simulink model "HighLevelLowLevel_Manual"  (R2023a)
settings: Solver=FixedStepAuto  StartTime=0.0  StopTime=25  FixedStep=0.0025  RelTol=1e-3
InitFcn:
  | startup
model workspace (MAT data in the model file):
  Cd = 2.24197803e-06
  Ct = 0.00010297
  Ixx = 113600
  Iyy = 113600
  Izz = 22620
  h = 0.05
values from neighbouring files (symbols this model uses):
  B_t = pinv(B)    [startup.m]
  g = 9.806    [startup.m]
  invI = I^-1    [startup.m]
  K_HL = round(K_HL, 6)    [startup.m]
  K_HL_FF = [K_HLtx(1,1), zeros(1,5), K_HLtx(1,2), zeros(1,5), K_HLtx(1,3), zeros(1,5) ... (first row only)    [startup.m]
  K_HL_manual = round(K_HL_manual, 6)    [startup.m]
  l = 0.053336    [startup.m]
  m = 6.2    [startup.m]
  sample_rate = 0.0025    [startup.m]
libraries: simulink_extras x12, matrix_library x8, aerolibanimutils x2, dspmtrx3 x2, shared6dof x1, commchan3 x1
settings Model: Creator=awahm  LastModifiedBy=lachlainm
settings DataIOCC: SaveFormat=StructureWithTime
settings OptimizationCC: DefaultParameterBehavior=Inlined  UseDivisionForNetSlopeComputation=on  GainParamInheritBuiltInType=on  UseFloatMulNetSlope=on  OptimizeBlockIOStorage=off  ZeroExternalMemoryAtStartup=off  ZeroInternalMemoryAtStartup=off  LifeSpan=1  OptimizeDataStoreBuffers=off  BusAssignmentInplaceUpdate=off
settings DebuggingCC: SFUnexpectedBacktrackingDiag=warning  SFNoUnconditionalDefaultTransitionDiag=warning
settings RTWCC: GenerateReport=on  BuildConfiguration=Debug  LaunchReport=on  TargetLang=C++
settings CodeAppCC: ForceParamTrailComments=on  MATLABSourceComments=on  EnableCustomComments=on
settings GRTTargetCC: TargetLangStandard=C++11 (ISO)  CombineSignalStateStructs=on  CodeInterfacePackaging=C++ class  SupportVariableSizeSignals=on  MultiInstanceErrorCode=Warning

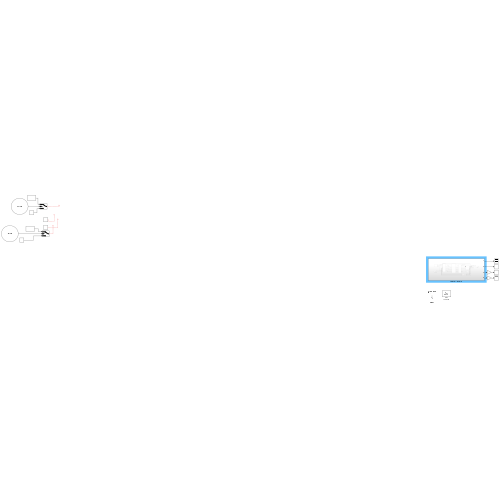
[thumbnail: Simulink's stored preview of the top-level diagram]
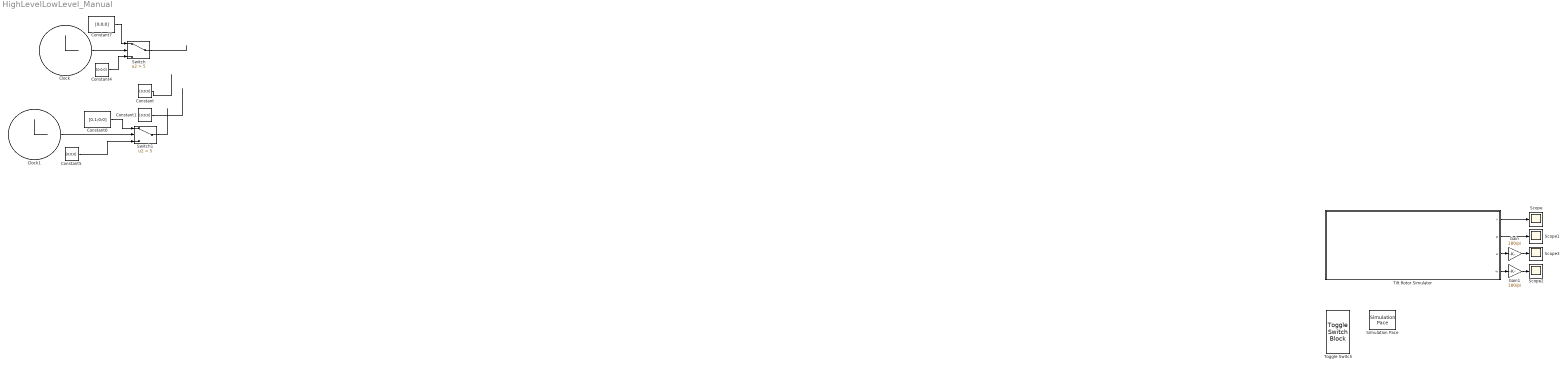
== system HighLevelLowLevel_Manual ==
  Clock : Clock
  Clock1 : Clock
  Constant{,1,4..5,7} (5 alike) : Constant  Value=[0;0;0]
  Constant6 : Constant  Value=[0.1;0;0]
  Gain : Gain  Gain=180/pi
  Gain1 : Gain  Gain=180/pi
  Scope{,1..3} (4 alike) : Scope
  Simulation Pace : aerolibanimutils/Simulation Pace  SimulationPace=1  SleepMode=Auto  OutputPaceError=off  SampleTime=sample_rate
  Switch : Switch  Criteria=u2 > Threshold  Threshold=5  SaturateOnIntegerOverflow=off  InputSameDT=off
  Switch1 : Switch  Criteria=u2 > Threshold  Threshold=5  SaturateOnIntegerOverflow=off  InputSameDT=off
  Tilt Rotor Simulator : Subsystem
  Toggle Switch : ToggleSwitchBlock
      settings: Values={{'Manual', 'Autonomous'}, [0 1]}
  wires:
  Constant/1 -> ?
  Switch1/1 -> ?
  Constant1/1 -> ?
  Clock/1 -> Switch/2
  Constant7/1 -> Switch/1
  Switch/1 -> ?
  Constant4/1 -> Switch/3
  Clock1/1 -> Switch1/2
  Constant6/1 -> Switch1/1
  Constant5/1 -> Switch1/3
  Tilt Rotor Simulator/1(v) -> Scope/1
  Tilt Rotor Simulator/4(w) -> Gain1/1
  Tilt Rotor Simulator/3(a) -> Gain/1
  Tilt Rotor Simulator/2(p) -> Scope1/1
  Gain/1 -> Scope3/1
  Gain1/1 -> Scope2/1

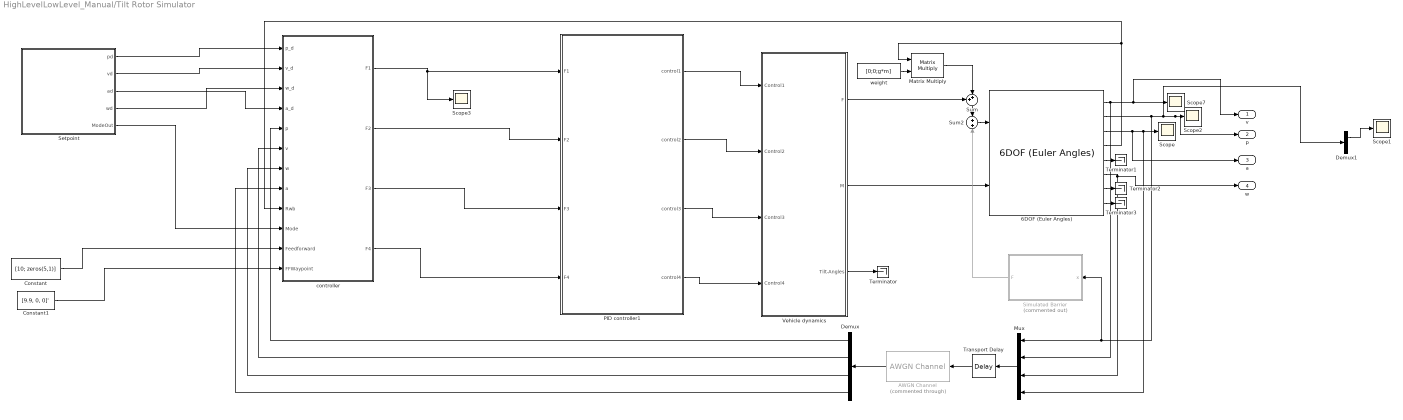
== system HighLevelLowLevel_Manual/Tilt Rotor Simulator ==
  6DOF (Euler Angles) : shared6dof/6DOF (Euler Angles)  units=Metric (MKS)  mtype=Fixed  rep=Euler Angles  xme_0=[0 0 0]  Vm_0=[0 0 0]  eul_0=[0 0 0]  pm_0=[0 0 0]  mass_0=6.2  mass_e=0.5  mass_f=2.0  inertia=I  inertia_e=eye(3)  inertia_f=2*eye(3)  k_quat=1.0  vre_flag=on  abi_flag=off  aMode=0  xme_statename=''  Vm_statename=''  eul_statename=''  quat_statename=''  pm_statename=''  mass_statename=''
  AWGN Channel : commchan3/AWGN Channel  Commented=through  LegacyMode=on  NoiseMethod="Signal to noise ratio  (SNR)"  noiseMode="Signal to noise ratio  (SNR)"  EbNo=10  EsNo=10  SNR=10  BitsPerSymbol=1  SignalPower=1  SamplesPerSymbol=1  SymbolPeriod=1  VarianceSource=Parameter  Variance=1  RandomStream=Global stream  Seed=67  SimulateUsing=Code generation
  Constant : Constant  Value=[10; zeros(5,1)]
  Constant1 : Constant  Value=[9.9, 0, 0]'
  Demux : Demux
  Demux1 : Demux  Outputs=3
  Matrix Multiply : Product  Multiplication=Matrix(*)
  Mux : Mux
  PID controller1 : Subsystem
  Scope{,1..3,7} (5 alike) : Scope
  Setpoint : Subsystem
  Simulated Barrier : MATLAB Function  Commented=on  TreatAsAtomicUnit=on  mask{x1=[10; -5], x2=[10; 5], E=1000000, thickness=0.1, A=0.5^2}
  Sum : Sum  Inputs=++|
  Sum2 : Sum  Inputs=+|+
  Terminator{,1..3} (4 alike) : Terminator
  Transport Delay : TransportDelay  DelayTime=0.006
  Vehicle dynamics : Subsystem
  controller : Subsystem  TreatAsAtomicUnit=on
  weight : Constant  Value=[0;0;g*m]
  v : Outport
  p : Outport  Port=2
  a : Outport  Port=3
  w : Outport  Port=4
  wires:
  6DOF (Euler Angles)/2 -> Demux1/1, p/1, Scope2/1, Simulated Barrier/1(x), Mux/1
  Mux/1 -> Transport Delay/1
  PID controller1/3(control3) -> Vehicle dynamics/3(Control3)
  6DOF (Euler Angles)/6 -> w/1, Mux/3
  weight/1 -> Matrix Multiply/2
  controller/4(F4) -> PID controller1/4(F4)
  Matrix Multiply/1 -> Sum/2
  Demux/1 -> controller/5(p)
  controller/1(F1) -> Scope3/1, PID controller1/1(F1)
  Demux/4 -> controller/8(a)
  Setpoint/1(pd) -> controller/1(p_d)
  PID controller1/1(control1) -> Vehicle dynamics/1(Control1)
  Vehicle dynamics/1(F) -> Sum/1
  controller/3(F3) -> PID controller1/3(F3)
  6DOF (Euler Angles)/8 -> Terminator3/1
  PID controller1/4(control4) -> Vehicle dynamics/4(Control4)
  Vehicle dynamics/3(Tilt-Angles) -> Terminator/1
  controller/2(F2) -> PID controller1/2(F2)
  Vehicle dynamics/2(M) -> 6DOF (Euler Angles)/2
  AWGN Channel/1 -> Demux/1
  6DOF (Euler Angles)/1 -> v/1, Scope7/1, Mux/2
  6DOF (Euler Angles)/3 -> a/1, Mux/4, Scope/1
  Setpoint/2(vd) -> controller/2(v_d)
  Demux/3 -> controller/7(w)
  PID controller1/2(control2) -> Vehicle dynamics/2(Control2)
  6DOF (Euler Angles)/7 -> Terminator2/1
  Demux/2 -> controller/6(v)
  Transport Delay/1 -> AWGN Channel/1
  6DOF (Euler Angles)/4 -> controller/9(Rwb), Matrix Multiply/1
  Setpoint/4(wd) -> controller/3(w_d)
  Setpoint/3(ad) -> controller/4(a_d)
  6DOF (Euler Angles)/5 -> Terminator1/1
  Sum/1 -> Sum2/1
  Sum2/1 -> 6DOF (Euler Angles)/1
  Simulated Barrier/1(F) -> Sum2/2
  Setpoint/5(ModeOut) -> controller/10(Mode)
  Constant/1 -> controller/11(Feedforward)
  Constant1/1 -> controller/12(FFWaypoint)
  Demux1/1 -> Scope1/1

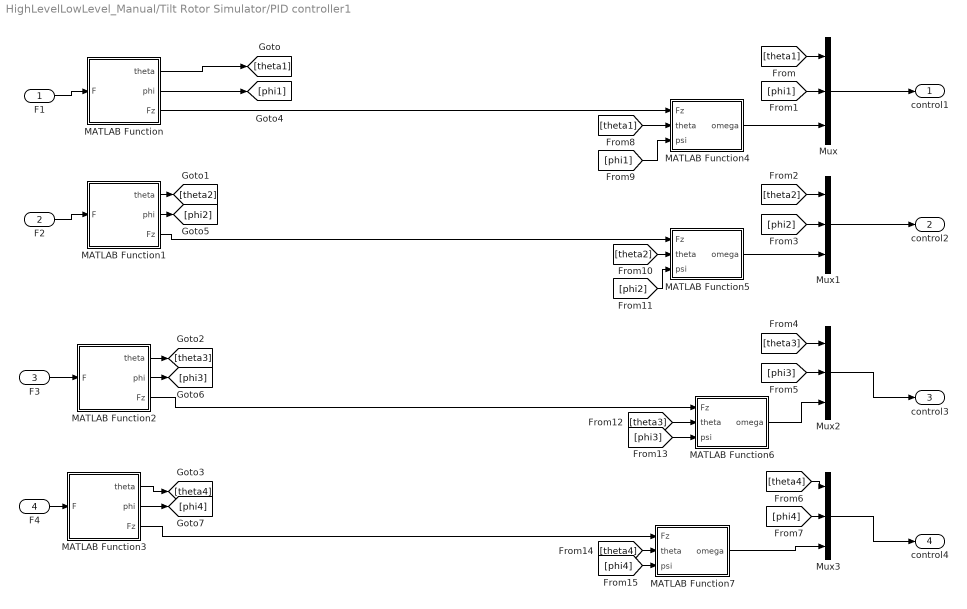
== system HighLevelLowLevel_Manual/Tilt Rotor Simulator/PID controller1 ==
  F1 : Inport
  F2 : Inport  Port=2
  F3 : Inport  Port=3
  F4 : Inport  Port=4
  MATLAB Function : MATLAB Function  TreatAsAtomicUnit=on
  MATLAB Function1 : MATLAB Function  TreatAsAtomicUnit=on
  MATLAB Function2 : MATLAB Function  TreatAsAtomicUnit=on
  MATLAB Function3 : MATLAB Function  TreatAsAtomicUnit=on
  MATLAB Function4 : MATLAB Function  TreatAsAtomicUnit=on
  MATLAB Function5 : MATLAB Function  TreatAsAtomicUnit=on
  MATLAB Function6 : MATLAB Function  TreatAsAtomicUnit=on
  MATLAB Function7 : MATLAB Function  TreatAsAtomicUnit=on
  Mux{,1..3} (4 alike) : Mux  Inputs=3
  control1 : Outport
  control2 : Outport  Port=2
  control3 : Outport  Port=3
  control4 : Outport  Port=4
  wires:
  Mux/1 -> control1/1
  MATLAB Function1/3(Fz) -> MATLAB Function5/1(Fz)
  [theta1] -> MATLAB Function4/2(theta)
  [phi2] -> MATLAB Function5/3(psi)
  MATLAB Function1/2(phi) -> [phi2]
  [theta3] -> MATLAB Function6/2(theta)
  MATLAB Function/3(Fz) -> MATLAB Function4/1(Fz)
  MATLAB Function3/2(phi) -> [phi4]
  [phi4] -> Mux3/2
  Mux2/1 -> control3/1
  MATLAB Function3/1(theta) -> [theta4]
  [phi3] -> MATLAB Function6/3(psi)
  MATLAB Function5/1(omega) -> Mux1/3
  [theta2] -> MATLAB Function5/2(theta)
  [theta1] -> Mux/1
  MATLAB Function7/1(omega) -> Mux3/3
  Mux1/1 -> control2/1
  MATLAB Function1/1(theta) -> [theta2]
  MATLAB Function4/1(omega) -> Mux/3
  [theta3] -> Mux2/1
  F2/1 -> MATLAB Function1/1(F)
  [phi4] -> MATLAB Function7/3(psi)
  MATLAB Function3/3(Fz) -> MATLAB Function7/1(Fz)
  [theta2] -> Mux1/1
  [phi2] -> Mux1/2
  MATLAB Function2/3(Fz) -> MATLAB Function6/1(Fz)
  [theta4] -> Mux3/1
  MATLAB Function2/2(phi) -> [phi3]
  Mux3/1 -> control4/1
  [phi3] -> Mux2/2
  F1/1 -> MATLAB Function/1(F)
  [phi1] -> Mux/2
  [phi1] -> MATLAB Function4/3(psi)
  F3/1 -> MATLAB Function2/1(F)
  MATLAB Function6/1(omega) -> Mux2/3
  MATLAB Function/1(theta) -> [theta1]
  MATLAB Function/2(phi) -> [phi1]
  [theta4] -> MATLAB Function7/2(theta)
  MATLAB Function2/1(theta) -> [theta3]
  F4/1 -> MATLAB Function3/1(F)

== system HighLevelLowLevel_Manual/Tilt Rotor Simulator/Setpoint ==
  Autonomous : Subsystem  VariantControl=auto
  Manual : Subsystem  VariantControl=manual
  Mode : Constant
  Switch{,1..3} (4 alike) : Switch  Criteria=u2 ~= 0  SaturateOnIntegerOverflow=off  InputSameDT=off
  pd : Outport
  vd : Outport  Port=2
  ad : Outport  Port=3
  wd : Outport  Port=4
  ModeOut : Outport  Port=5
  wires:
  Autonomous/1(pd) -> Switch/1
  Autonomous/2(vd) -> Switch1/1
  Autonomous/3(ad) -> Switch2/1
  Autonomous/4(wd) -> Switch3/1
  Manual/1(pd) -> Switch/3
  Manual/2(vd) -> Switch1/3
  Manual/3(wd) -> Switch3/3
  Manual/4(ad) -> Switch2/3
  Switch3/1 -> wd/1
  Switch2/1 -> ad/1
  Switch1/1 -> vd/1
  Switch/1 -> pd/1
  Mode/1 -> ModeOut/1, Switch/2, Switch3/2, Switch2/2, Switch1/2

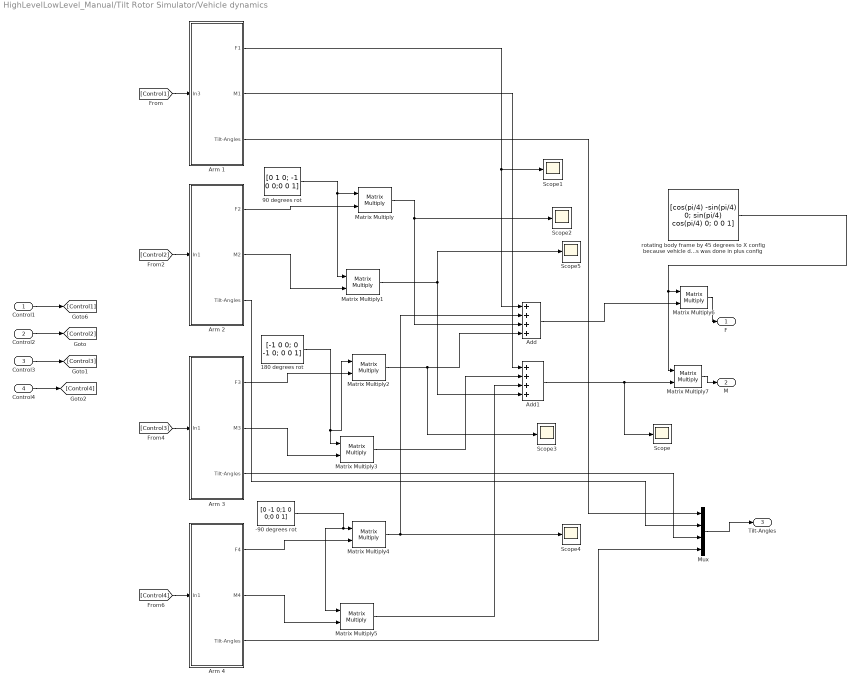
== system HighLevelLowLevel_Manual/Tilt Rotor Simulator/Vehicle dynamics ==
  Control1 : Inport
  Control2 : Inport  Port=2
  Control3 : Inport  Port=3
  Control4 : Inport  Port=4
  -90 degrees rot : Constant  Value=[0 -1 0;1 0 0;0 0 1]
  180 degrees rot : Constant  Value=[-1 0 0; 0 -1 0; 0 0 1]
  90 degrees rot : Constant  Value=[0 1 0; -1 0 0;0 0 1]
  Add : Sum  Inputs=++++
  Add1 : Sum  Inputs=++++
  Arm 1 : Subsystem
  Arm 2 : Subsystem
  Arm 3 : Subsystem
  Arm 4 : Subsystem
  Matrix Multiply{,1..7} (8 alike) : Product  Multiplication=Matrix(*)
  Mux : Mux
  Scope{,1..5} (6 alike) : Scope
  rotating body frame by 45 degrees to X config because vehicle dynamics was done in plus config : Constant  Value=|
      | [cos(pi/4) -sin(pi/4) 0;
      | sin(pi/4) cos(pi/4) 0;
      | 0 0 1]
  F : Outport
  M : Outport  Port=2
  Tilt-Angles : Outport  Port=3
  wires:
  Control1/1 -> [Control1]
  Control2/1 -> [Control2]
  Control3/1 -> [Control3]
  Control4/1 -> [Control4]
  [Control1] -> Arm 1/1(In3)
  Arm 1/1(F1) -> Add/1, Scope1/1
  Arm 1/2(M1) -> Add1/1
  90 degrees rot/1 -> Matrix Multiply1/1, Matrix Multiply/1
  Arm 2/1(F2) -> Matrix Multiply/2
  Matrix Multiply/1 -> Scope2/1, Add/3
  Arm 2/2(M2) -> Matrix Multiply1/2
  Matrix Multiply1/1 -> Add1/4, Scope5/1
  [Control2] -> Arm 2/1(In1)
  -90 degrees rot/1 -> Matrix Multiply5/1, Matrix Multiply4/1
  Arm 3/1(F3) -> Matrix Multiply2/2
  Matrix Multiply3/1 -> Add1/2
  [Control3] -> Arm 3/1(In1)
  Arm 3/2(M3) -> Matrix Multiply3/2
  180 degrees rot/1 -> Matrix Multiply3/1, Matrix Multiply2/1
  Arm 4/2(M4) -> Matrix Multiply5/2
  Arm 4/1(F4) -> Matrix Multiply4/2
  Matrix Multiply5/1 -> Add1/3
  [Control4] -> Arm 4/1(In1)
  Matrix Multiply2/1 -> Scope3/1, Add/4
  Matrix Multiply4/1 -> Add/2, Scope4/1
  rotating body frame by 45 degrees to X config because vehicle dynamics was done in plus config/1 -> Matrix Multiply6/1, Matrix Multiply7/1
  Add/1 -> Matrix Multiply6/2
  Add1/1 -> Matrix Multiply7/2, Scope/1
  Matrix Multiply7/1 -> M/1
  Matrix Multiply6/1 -> F/1
  Arm 1/3(Tilt-Angles) -> Mux/1
  Arm 2/3(Tilt-Angles) -> Mux/2
  Arm 3/3(Tilt-Angles) -> Mux/3
  Arm 4/3(Tilt-Angles) -> Mux/4
  Mux/1 -> Tilt-Angles/1

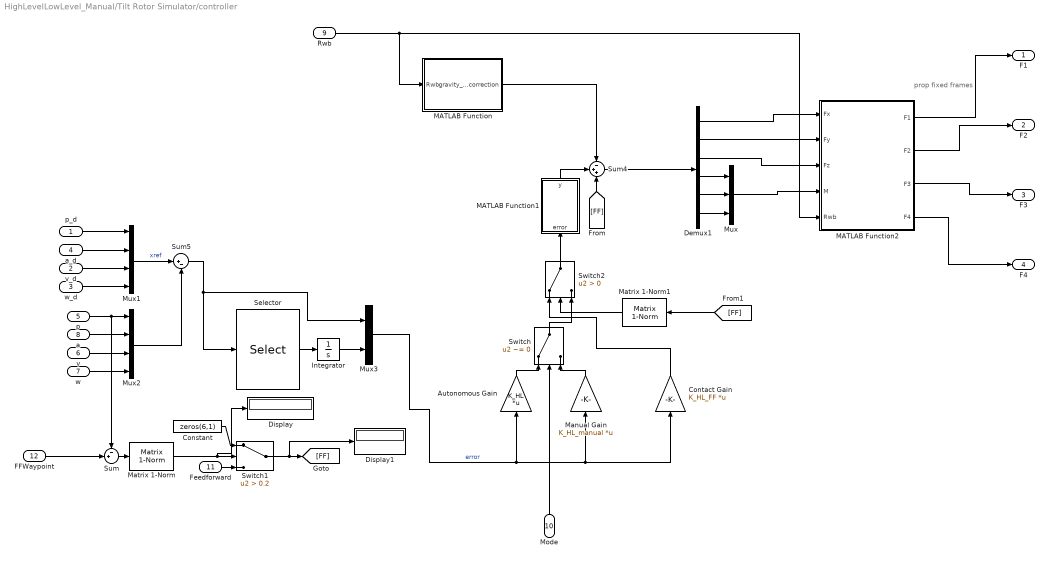
== system HighLevelLowLevel_Manual/Tilt Rotor Simulator/controller ==
  note: prop fixed frames
  p_d : Inport
  v_d : Inport  Port=2
  w_d : Inport  Port=3
  a_d : Inport  Port=4
  p : Inport  Port=5
  v : Inport  Port=6
  w : Inport  Port=7
  a : Inport  Port=8
  Rwb : Inport  Port=9
  Mode : Inport  Port=10
  Feedforward : Inport  Port=11
  FFWaypoint : Inport  Port=12
  Autonomous Gain : Gain  Gain=K_HL  Multiplication=Matrix(K*u) (u vector)
  Constant : Constant  Value=zeros(6,1)
  Contact Gain : Gain  Gain=K_HL_FF  Multiplication=Matrix(K*u) (u vector)
  Demux1 : Demux  Outputs=6
  Display : Display
  Display1 : Display
  Integrator : Integrator  LimitOutput=on  UpperSaturationLimit=0.05  LowerSaturationLimit=-0.05
  MATLAB Function : MATLAB Function  TreatAsAtomicUnit=on  mask{invI=invI, l=l, g=g, B_t=B_t}
  MATLAB Function1 : MATLAB Function  TreatAsAtomicUnit=on
  MATLAB Function2 : MATLAB Function  TreatAsAtomicUnit=on
  Manual Gain : Gain  Gain=K_HL_manual  Multiplication=Matrix(K*u) (u vector)
  Matrix 1-Norm : dspmtrx3/Matrix  1-Norm  roundingMode=Floor  overflowMode=off  outputDataTypeStr=Inherit: Same as accumulator  outputMin=[]  outputMax=[]  outputLastDataTypeStr=Inherit: Same as accumulator
  Matrix 1-Norm1 : dspmtrx3/Matrix  1-Norm  roundingMode=Floor  overflowMode=off  outputDataTypeStr=Inherit: Same as accumulator  outputMin=[]  outputMax=[]  outputLastDataTypeStr=Inherit: Same as accumulator
  Mux : Mux  Inputs=3
  Mux1 : Mux
  Mux2 : Mux
  Mux3 : Mux  Inputs=2
  Selector : Selector  InputPortWidth=12  IndexOptions=Index vector (dialog)  Indices=[1 2 3 4 5 6]  OutputSizes=1
  Sum : Sum  Inputs=-+|
  Sum4 : Sum  Inputs=-++
  Sum5 : Sum  Inputs=|+-
  Switch : Switch  Criteria=u2 ~= 0  SaturateOnIntegerOverflow=off  InputSameDT=off
  Switch1 : Switch  Criteria=u2 > Threshold  Threshold=0.2  SaturateOnIntegerOverflow=off  InputSameDT=off
  Switch2 : Switch  Criteria=u2 > Threshold  SaturateOnIntegerOverflow=off  InputSameDT=off
  F1 : Outport
  F2 : Outport  Port=2
  F3 : Outport  Port=3
  F4 : Outport  Port=4
  wires:
  MATLAB Function2/3(F3) -> F3/1
  p/1 -> Sum/1, Mux2/1
  Demux1/5 -> Mux/2
  w_d/1 -> Mux1/4
  Demux1/6 -> Mux/3
  a_d/1 -> Mux1/2
  Demux1/4 -> Mux/1
  MATLAB Function2/1(F1) -> F1/1
  a/1 -> Mux2/2
  MATLAB Function2/4(F4) -> F4/1
  Mux/1 -> MATLAB Function2/4(M)
  Demux1/1 -> MATLAB Function2/1(Fx)
  Mux1/1 -> Sum5/1  "xref"
  p_d/1 -> Mux1/1
  Sum5/1 -> Mux3/1, Selector/1
  MATLAB Function2/2(F2) -> F2/1
  v_d/1 -> Mux1/3
  Demux1/2 -> MATLAB Function2/2(Fy)
  w/1 -> Mux2/4
  Integrator/1 -> Mux3/2
  v/1 -> Mux2/3
  Sum4/1 -> Demux1/1
  Selector/1 -> Integrator/1
  MATLAB Function/1(gravity_correction) -> Sum4/1
  Rwb/1 -> MATLAB Function/1(Rwb), MATLAB Function2/5(Rwb)
  Demux1/3 -> MATLAB Function2/3(Fz)
  MATLAB Function1/1(y) -> Sum4/2
  Mux3/1 -> Contact Gain/1, Manual Gain/1, Autonomous Gain/1  "error"
  Mux2/1 -> Sum5/2
  Switch/1 -> Switch2/3
  Autonomous Gain/1 -> Switch/1
  Manual Gain/1 -> Switch/3
  Mode/1 -> Switch/2
  Feedforward/1 -> Switch1/3
  [FF] -> Sum4/3
  FFWaypoint/1 -> Sum/2
  Sum/1 -> Matrix 1-Norm/1
  Constant/1 -> Switch1/1
  Switch1/1 -> Display1/1, [FF]
  Switch2/1 -> MATLAB Function1/1(error)
  Matrix 1-Norm/1 -> Display/1, Switch1/2
  [FF] -> Matrix 1-Norm1/1
  Matrix 1-Norm1/1 -> Switch2/2
  Contact Gain/1 -> Switch2/1

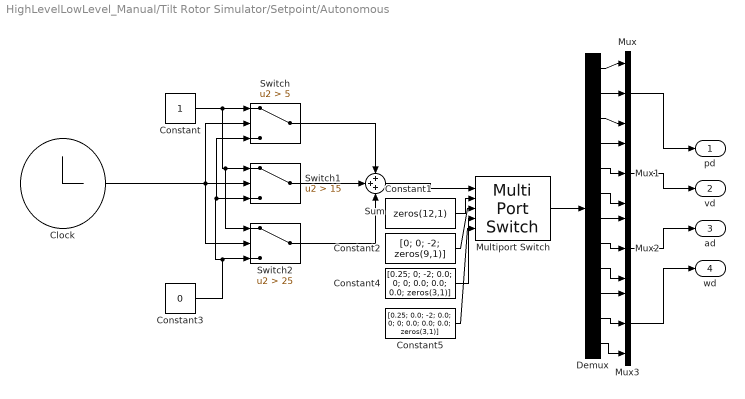
== system HighLevelLowLevel_Manual/Tilt Rotor Simulator/Setpoint/Autonomous ==
  Clock : Clock
  Constant : Constant
  Constant1 : Constant  Value=zeros(12,1)
  Constant2 : Constant  Value=[0; 0; -2; zeros(9,1)]
  Constant3 : Constant  Value=0
  Constant4 : Constant  Value=[0.25; 0; -2; 0.0; 0; 0; 0.0; 0.0; 0.0; zeros(3,1)]
  Constant5 : Constant  Value=[0.25; 0.0; -2; 0.0; 0; 0; 0.0; 0.0; 0.0; zeros(3,1)]
  Demux : Demux  Outputs=12
  Multiport Switch : MultiPortSwitch  DataPortOrder=Zero-based contiguous  Inputs=4  zeroidx=on  SaturateOnIntegerOverflow=off  InputSameDT=off
  Mux{,1..3} (4 alike) : Mux  Inputs=3
  Sum : Sum  Inputs=+++
  Switch : Switch  Criteria=u2 > Threshold  Threshold=5  SaturateOnIntegerOverflow=off  InputSameDT=off
  Switch1 : Switch  Criteria=u2 > Threshold  Threshold=15  SaturateOnIntegerOverflow=off  InputSameDT=off
  Switch2 : Switch  Criteria=u2 > Threshold  Threshold=25  SaturateOnIntegerOverflow=off  InputSameDT=off
  pd : Outport
  vd : Outport  Port=2
  ad : Outport  Port=3
  wd : Outport  Port=4
  wires:
  Demux/1 -> Mux/1
  Demux/2 -> Mux/2
  Demux/3 -> Mux/3
  Demux/4 -> Mux1/1
  Demux/5 -> Mux1/2
  Demux/6 -> Mux1/3
  Demux/8 -> Mux2/2
  Demux/7 -> Mux2/1
  Demux/9 -> Mux2/3
  Demux/11 -> Mux3/2
  Demux/10 -> Mux3/1
  Demux/12 -> Mux3/3
  Mux/1 -> pd/1
  Mux1/1 -> vd/1
  Mux2/1 -> ad/1
  Mux3/1 -> wd/1
  Multiport Switch/1 -> Demux/1
  Clock/1 -> Switch2/2, Switch/2, Switch1/2
  Constant/1 -> Switch2/1, Switch1/1, Switch/1
  Constant3/1 -> Switch/3, Switch1/3, Switch2/3
  Switch1/1 -> Sum/2
  Switch/1 -> Sum/1
  Switch2/1 -> Sum/3
  Sum/1 -> Multiport Switch/1
  Constant1/1 -> Multiport Switch/2
  Constant2/1 -> Multiport Switch/3
  Constant4/1 -> Multiport Switch/4
  Constant5/1 -> Multiport Switch/5

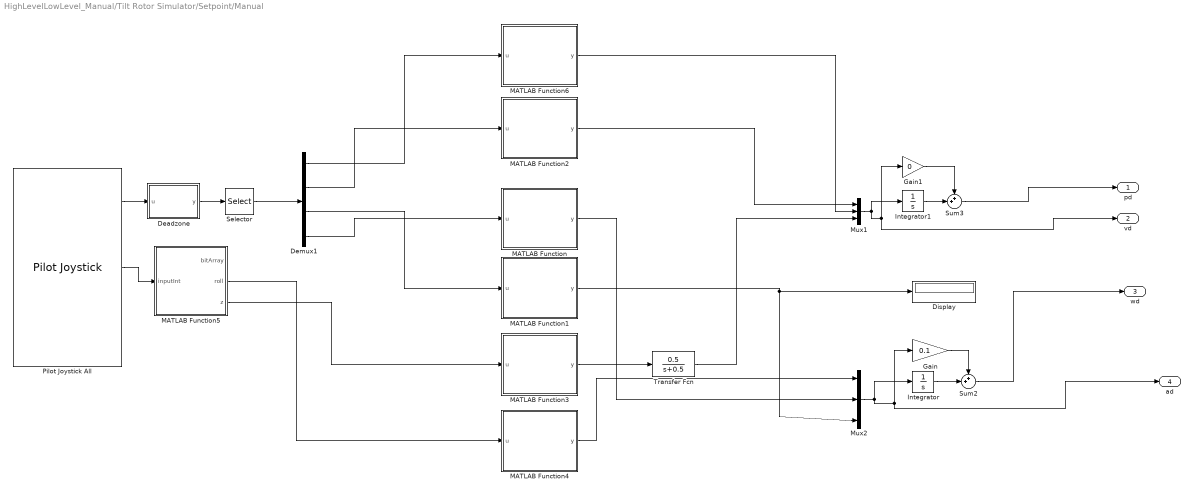
== system HighLevelLowLevel_Manual/Tilt Rotor Simulator/Setpoint/Manual ==
  Deadzone : MATLAB Function  TreatAsAtomicUnit=on
  Demux1 : Demux
  Display : Display
  Gain : Gain  Gain=0.1
  Gain1 : Gain  Gain=0
  Integrator : Integrator
  Integrator1 : Integrator
  MATLAB Function : MATLAB Function  TreatAsAtomicUnit=on  mask{min_in=-1, min_out=-0.0175 * 5, max_in=1, max_out=0.0175 * 5}
  MATLAB Function1 : MATLAB Function  TreatAsAtomicUnit=on  mask{min_in=0, min_out=-0.087, max_in=1, max_out=0.087}
  MATLAB Function2 : MATLAB Function  TreatAsAtomicUnit=on  mask{min_in=1, min_out=-5, max_in=-1, max_out=5}
  MATLAB Function3 : MATLAB Function  TreatAsAtomicUnit=on  mask{min_in=-1, min_out=-5, max_in=1, max_out=5}
  MATLAB Function4 : MATLAB Function  TreatAsAtomicUnit=on  mask{min_in=-1, min_out=-0.0175 * 5, max_in=1, max_out=0.0175 * 5}
  MATLAB Function5 : MATLAB Function  TreatAsAtomicUnit=on
  MATLAB Function6 : MATLAB Function  TreatAsAtomicUnit=on  mask{min_in=-1, min_out=-5, max_in=1, max_out=5}
  Mux1 : Mux  Inputs=3
  Mux2 : Mux  Inputs=3
  Pilot Joystick All : aerolibanimutils/Pilot Joystick  JoystickID=Joystick1  OutputConfiguration=AllOutputs  SampleTime=sample_rate
      settings: LibrarySourceBlock=aerolibanimutils/Pilot Joystick All
  Selector : Selector  InputPortWidth=6  IndexOptions=Index vector (dialog)  Indices=[1 2 3 4]  OutputSizes=1
  Sum2 : Sum  Inputs=++|
  Sum3 : Sum  Inputs=++|
  Transfer Fcn : TransferFcn  Numerator=[0.5]  Denominator=[1 0.5]
  pd : Outport
  vd : Outport  Port=2
  wd : Outport  Port=3
  ad : Outport  Port=4
  wires:
  Demux1/4 -> MATLAB Function/1(u)
  MATLAB Function/1(y) -> Mux2/2
  Demux1/1 -> MATLAB Function6/1(u)
  MATLAB Function2/1(y) -> Mux1/1
  Pilot Joystick All/1 -> Deadzone/1(u)
  Selector/1 -> Demux1/1
  Gain1/1 -> Sum3/1
  Pilot Joystick All/2 -> MATLAB Function5/1(inputInt)
  MATLAB Function4/1(y) -> Mux2/1
  MATLAB Function5/2(roll) -> MATLAB Function4/1(u)
  Mux2/1 -> Integrator/1, Gain/1, ad/1
  Integrator1/1 -> Sum3/2
  MATLAB Function1/1(y) -> Display/1, Mux2/3
  Gain/1 -> Sum2/1
  Demux1/2 -> MATLAB Function2/1(u)
  MATLAB Function3/1(y) -> Transfer Fcn/1
  MATLAB Function5/3(z) -> MATLAB Function3/1(u)
  MATLAB Function6/1(y) -> Mux1/2
  Deadzone/1(y) -> Selector/1
  Demux1/3 -> MATLAB Function1/1(u)
  Sum2/1 -> wd/1
  Transfer Fcn/1 -> Mux1/3
  Integrator/1 -> Sum2/2
  Mux1/1 -> vd/1, Gain1/1, Integrator1/1
  Sum3/1 -> pd/1

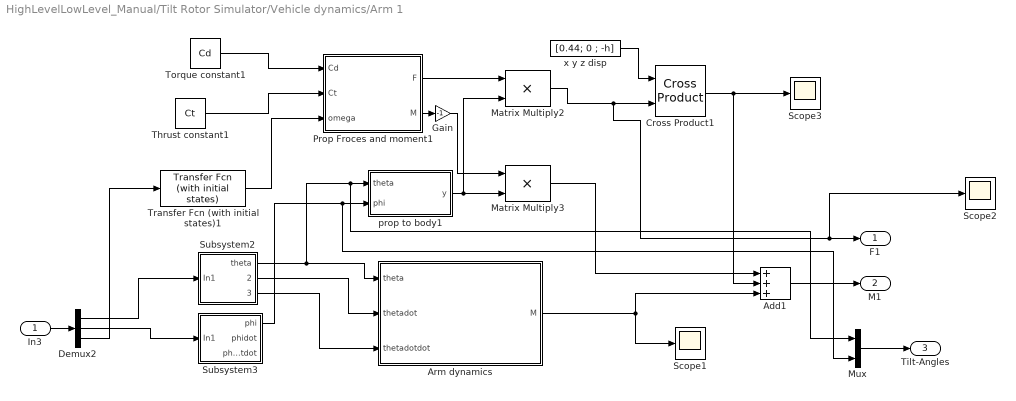
== system HighLevelLowLevel_Manual/Tilt Rotor Simulator/Vehicle dynamics/Arm 1 ==
  In3 : Inport
  Add1 : Sum  Inputs=+++
  Arm dynamics : Subsystem
  Cross Product1 : matrix_library/Cross Product
  Demux2 : Demux  Outputs=3
  Gain : Gain  Gain=-1
  Matrix Multiply2 : Product
  Matrix Multiply3 : Product
  Mux : Mux  Inputs=2
  Prop Froces and moment1 : Subsystem
  Scope1 : Scope
  Scope2 : Scope
  Scope3 : Scope
  Subsystem2 : Subsystem
  Subsystem3 : Subsystem
  Thrust constant1 : Constant  Value=Ct
  Torque constant1 : Constant  Value=Cd
  Transfer Fcn (with initial states)1 : simulink_extras/Additional Linear/Transfer Fcn (with initial states)  N=[153.35]  D=[1 20.06 153.35]  X0=0
  prop to body1 : MATLAB Function  TreatAsAtomicUnit=on
  x y z disp : Constant  Value=[0.44; 0 ; -h]
  F1 : Outport
  M1 : Outport  Port=2
  Tilt-Angles : Outport  Port=3
  wires:
  x y z disp/1 -> Cross Product1/1
  Subsystem2/2(thetadot) -> Arm dynamics/2(thetadot)
  Cross Product1/1 -> Add1/2, Scope3/1
  In3/1 -> Demux2/1
  Prop Froces and moment1/1(F) -> Matrix Multiply2/1
  Arm dynamics/1(M) -> Add1/3, Scope1/1
  Demux2/2 -> Subsystem3/1(In1)
  Thrust constant1/1 -> Prop Froces and moment1/2(Ct)
  Torque constant1/1 -> Prop Froces and moment1/1(Cd)
  Add1/1 -> M1/1
  Matrix Multiply3/1 -> Add1/1
  prop to body1/1(y) -> Matrix Multiply3/2, Matrix Multiply2/2
  Demux2/1 -> Subsystem2/1(In1)
  Subsystem2/1(theta) -> Arm dynamics/1(theta), Mux/1, prop to body1/1(theta)
  Matrix Multiply2/1 -> Cross Product1/2, Scope2/1, F1/1
  Subsystem3/1(phi) -> Mux/2, prop to body1/2(phi)
  Subsystem2/3(thetadotdot) -> Arm dynamics/3(thetadotdot)
  Demux2/3 -> Transfer Fcn (with initial states)1/1
  Transfer Fcn (with initial states)1/1 -> Prop Froces and moment1/3(omega)
  Mux/1 -> Tilt-Angles/1
  Prop Froces and moment1/2(M) -> Gain/1
  Gain/1 -> Matrix Multiply3/1

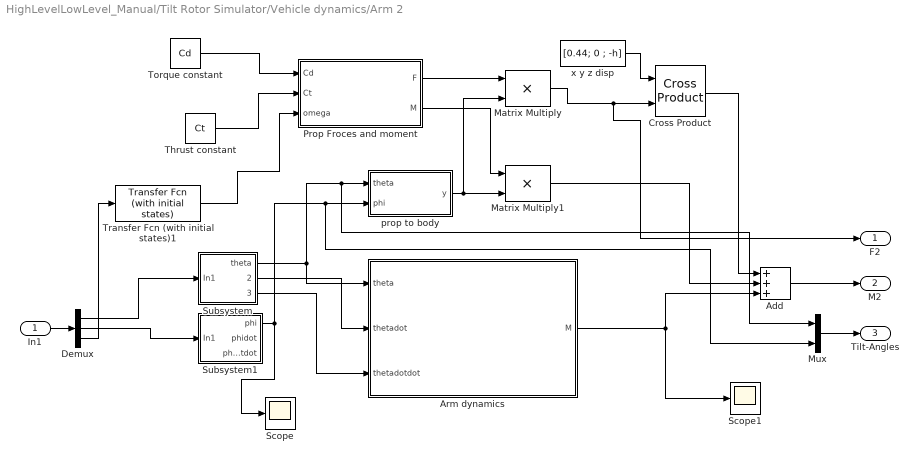
== system HighLevelLowLevel_Manual/Tilt Rotor Simulator/Vehicle dynamics/Arm 2 ==
  In1 : Inport
  Add : Sum  Inputs=+++
  Arm dynamics : Subsystem
  Cross Product : matrix_library/Cross Product
  Demux : Demux  Outputs=3
  Matrix Multiply : Product
  Matrix Multiply1 : Product
  Mux : Mux  Inputs=2
  Prop Froces and moment : Subsystem
  Scope : Scope
  Scope1 : Scope
  Subsystem : Subsystem
  Subsystem1 : Subsystem
  Thrust constant : Constant  Value=Ct
  Torque constant : Constant  Value=Cd
  Transfer Fcn (with initial states)1 : simulink_extras/Additional Linear/Transfer Fcn (with initial states)  N=[153.35]  D=[1 20.06 153.35]  X0=0
  prop to body : MATLAB Function  TreatAsAtomicUnit=on
  x y z disp : Constant  Value=[0.44; 0 ; -h]
  F2 : Outport
  M2 : Outport  Port=2
  Tilt-Angles : Outport  Port=3
  wires:
  prop to body/1(y) -> Matrix Multiply1/2, Matrix Multiply/2
  Demux/2 -> Subsystem1/1(In1)
  Matrix Multiply/1 -> Cross Product/2, F2/1
  Prop Froces and moment/1(F) -> Matrix Multiply/1
  Subsystem/1(theta) -> Arm dynamics/1(theta), Mux/1, prop to body/1(theta)
  Matrix Multiply1/1 -> Add/2
  Subsystem1/1(phi) -> Scope/1, Mux/2, prop to body/2(phi)
  Demux/1 -> Subsystem/1(In1)
  x y z disp/1 -> Cross Product/1
  Add/1 -> M2/1
  Torque constant/1 -> Prop Froces and moment/1(Cd)
  Thrust constant/1 -> Prop Froces and moment/2(Ct)
  Cross Product/1 -> Add/1
  In1/1 -> Demux/1
  Subsystem/2(thetadot) -> Arm dynamics/2(thetadot)
  Subsystem/3(thetadotdot) -> Arm dynamics/3(thetadotdot)
  Arm dynamics/1(M) -> Add/3, Scope1/1
  Demux/3 -> Transfer Fcn (with initial states)1/1
  Prop Froces and moment/2(M) -> Matrix Multiply1/1
  Transfer Fcn (with initial states)1/1 -> Prop Froces and moment/3(omega)
  Mux/1 -> Tilt-Angles/1

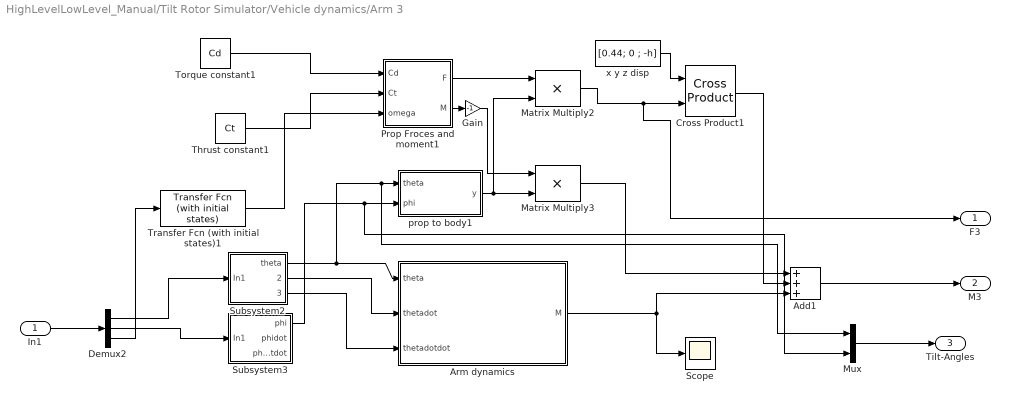
== system HighLevelLowLevel_Manual/Tilt Rotor Simulator/Vehicle dynamics/Arm 3 ==
  In1 : Inport
  Add1 : Sum  Inputs=+++
  Arm dynamics : Subsystem
  Cross Product1 : matrix_library/Cross Product
  Demux2 : Demux  Outputs=3
  Gain : Gain  Gain=-1
  Matrix Multiply2 : Product
  Matrix Multiply3 : Product
  Mux : Mux  Inputs=2
  Prop Froces and moment1 : Subsystem
  Scope : Scope
  Subsystem2 : Subsystem
  Subsystem3 : Subsystem
  Thrust constant1 : Constant  Value=Ct
  Torque constant1 : Constant  Value=Cd
  Transfer Fcn (with initial states)1 : simulink_extras/Additional Linear/Transfer Fcn (with initial states)  N=[153.35]  D=[1 20.06 153.35]  X0=0
  prop to body1 : MATLAB Function  TreatAsAtomicUnit=on
  x y z disp : Constant  Value=[0.44; 0 ; -h]
  F3 : Outport
  M3 : Outport  Port=2
  Tilt-Angles : Outport  Port=3
  wires:
  x y z disp/1 -> Cross Product1/1
  Subsystem2/2(thetadot) -> Arm dynamics/2(thetadot)
  Cross Product1/1 -> Add1/2
  In1/1 -> Demux2/1
  Prop Froces and moment1/1(F) -> Matrix Multiply2/1
  Arm dynamics/1(M) -> Add1/3, Scope/1
  Demux2/2 -> Subsystem3/1(In1)
  Thrust constant1/1 -> Prop Froces and moment1/2(Ct)
  Torque constant1/1 -> Prop Froces and moment1/1(Cd)
  Add1/1 -> M3/1
  Matrix Multiply3/1 -> Add1/1
  prop to body1/1(y) -> Matrix Multiply3/2, Matrix Multiply2/2
  Demux2/1 -> Subsystem2/1(In1)
  Subsystem2/1(theta) -> Arm dynamics/1(theta), Mux/1, prop to body1/1(theta)
  Demux2/3 -> Transfer Fcn (with initial states)1/1
  Matrix Multiply2/1 -> Cross Product1/2, F3/1
  Subsystem3/1(phi) -> Mux/2, prop to body1/2(phi)
  Subsystem2/3(thetadotdot) -> Arm dynamics/3(thetadotdot)
  Transfer Fcn (with initial states)1/1 -> Prop Froces and moment1/3(omega)
  Mux/1 -> Tilt-Angles/1
  Prop Froces and moment1/2(M) -> Gain/1
  Gain/1 -> Matrix Multiply3/1

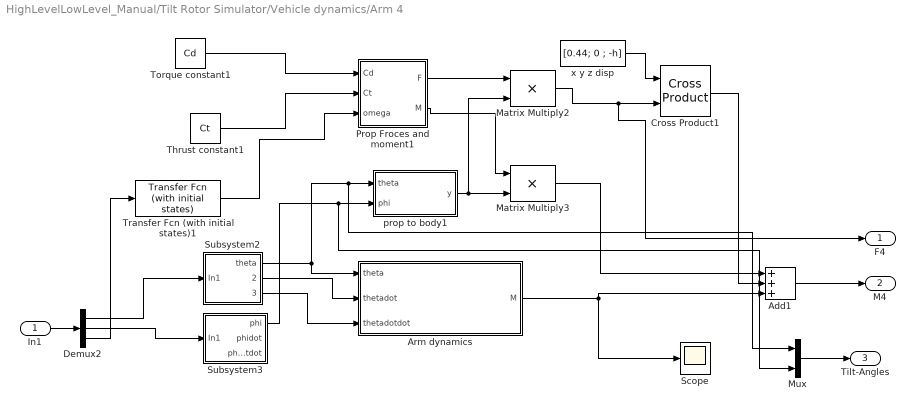
== system HighLevelLowLevel_Manual/Tilt Rotor Simulator/Vehicle dynamics/Arm 4 ==
  In1 : Inport
  Add1 : Sum  Inputs=+++
  Arm dynamics : Subsystem
  Cross Product1 : matrix_library/Cross Product
  Demux2 : Demux  Outputs=3
  Matrix Multiply2 : Product
  Matrix Multiply3 : Product
  Mux : Mux  Inputs=2
  Prop Froces and moment1 : Subsystem
  Scope : Scope
  Subsystem2 : Subsystem
  Subsystem3 : Subsystem
  Thrust constant1 : Constant  Value=Ct
  Torque constant1 : Constant  Value=Cd
  Transfer Fcn (with initial states)1 : simulink_extras/Additional Linear/Transfer Fcn (with initial states)  N=[153.35]  D=[1 20.06 153.35]  X0=0
  prop to body1 : MATLAB Function  TreatAsAtomicUnit=on
  x y z disp : Constant  Value=[0.44; 0 ; -h]
  F4 : Outport
  M4 : Outport  Port=2
  Tilt-Angles : Outport  Port=3
  wires:
  x y z disp/1 -> Cross Product1/1
  Subsystem2/2(thetadot) -> Arm dynamics/2(thetadot)
  Cross Product1/1 -> Add1/2
  In1/1 -> Demux2/1
  Prop Froces and moment1/1(F) -> Matrix Multiply2/1
  Arm dynamics/1(M) -> Add1/3, Scope/1
  Demux2/2 -> Subsystem3/1(In1)
  Thrust constant1/1 -> Prop Froces and moment1/2(Ct)
  Torque constant1/1 -> Prop Froces and moment1/1(Cd)
  Add1/1 -> M4/1
  Matrix Multiply3/1 -> Add1/1
  prop to body1/1(y) -> Matrix Multiply3/2, Matrix Multiply2/2
  Demux2/1 -> Subsystem2/1(In1)
  Subsystem2/1(theta) -> Arm dynamics/1(theta), Mux/1, prop to body1/1(theta)
  Matrix Multiply2/1 -> Cross Product1/2, F4/1
  Subsystem3/1(phi) -> Mux/2, prop to body1/2(phi)
  Subsystem2/3(thetadotdot) -> Arm dynamics/3(thetadotdot)
  Demux2/3 -> Transfer Fcn (with initial states)1/1
  Prop Froces and moment1/2(M) -> Matrix Multiply3/1
  Transfer Fcn (with initial states)1/1 -> Prop Froces and moment1/3(omega)
  Mux/1 -> Tilt-Angles/1

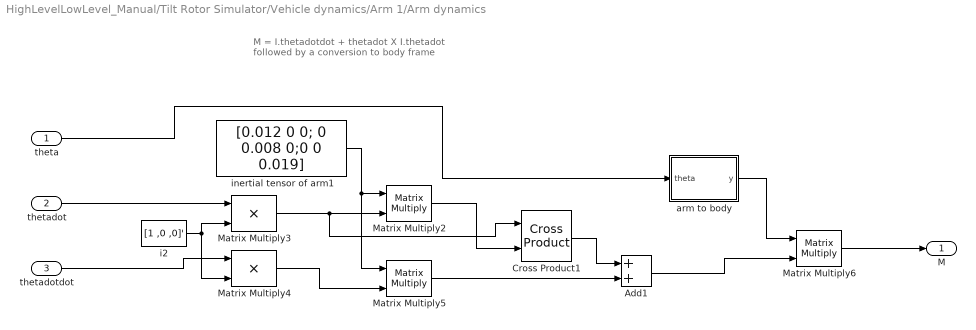
== system HighLevelLowLevel_Manual/Tilt Rotor Simulator/Vehicle dynamics/Arm 1/Arm dynamics ==
  note: M = I.thetadotdot + thetadot X I.thetadot
      | followed by a conversion to body frame
  theta : Inport
  thetadot : Inport  Port=2
  thetadotdot : Inport  Port=3
  Add1 : Sum
  Cross Product1 : matrix_library/Cross Product
  Matrix Multiply2 : Product  Multiplication=Matrix(*)
  Matrix Multiply3 : Product
  Matrix Multiply4 : Product
  Matrix Multiply5 : Product  Multiplication=Matrix(*)
  Matrix Multiply6 : Product  Multiplication=Matrix(*)
  arm to body : MATLAB Function  TreatAsAtomicUnit=on
  i2 : Constant  Value=[1 ,0 ,0]'
  inertial tensor of arm1 : Constant  Value=[0.012 0 0; 0 0.008 0;0 0 0.019]
  M : Outport
  wires:
  Matrix Multiply3/1 -> Cross Product1/1, Matrix Multiply2/2
  inertial tensor of arm1/1 -> Matrix Multiply5/1, Matrix Multiply2/1
  thetadotdot/1 -> Matrix Multiply4/1
  Matrix Multiply4/1 -> Matrix Multiply5/2
  Matrix Multiply5/1 -> Add1/2
  i2/1 -> Matrix Multiply4/2, Matrix Multiply3/2
  arm to body/1(y) -> Matrix Multiply6/1
  Matrix Multiply2/1 -> Cross Product1/2
  Cross Product1/1 -> Add1/1
  Add1/1 -> Matrix Multiply6/2
  thetadot/1 -> Matrix Multiply3/1
  Matrix Multiply6/1 -> M/1
  theta/1 -> arm to body/1(theta)

== system HighLevelLowLevel_Manual/Tilt Rotor Simulator/Vehicle dynamics/Arm 1/Prop Froces and moment1 ==
  note: T = Ctx w^2
      | Q = Cd x w^2
  Cd : Inport
  Ct : Inport  Port=2
  omega : Inport  Port=3
  Gain : Gain  Gain=-1
  Product{,1..3} (4 alike) : Product
  F : Outport
  M : Outport  Port=2
  wires:
  omega/1 -> Product3/1, Product2/2, Product1/2, Product/2
  Ct/1 -> Product2/1
  Product2/1 -> Product3/2
  Product3/1 -> Gain/1
  Product/1 -> Product1/1
  Product1/1 -> M/1
  Cd/1 -> Product/1
  Gain/1 -> F/1

== system HighLevelLowLevel_Manual/Tilt Rotor Simulator/Vehicle dynamics/Arm 1/Subsystem2 ==
  In1 : Inport
  Derivative : Derivative
  Derivative1 : Derivative  CoefficientInTFapproximation=1
  Scope : Scope
  Scope1 : Scope
  Scope2 : Scope
  Transfer Fcn (with initial states)1 : simulink_extras/Additional Linear/Transfer Fcn (with initial states)  N=[153.5000]  D="[1  20.06  153.3]"  X0=0
  theta : Outport
  thetadot : Outport  Port=2
  thetadotdot : Outport  Port=3
  wires:
  Derivative/1 -> Scope2/1, thetadot/1, Derivative1/1
  Transfer Fcn (with initial states)1/1 -> Derivative/1, Scope/1, theta/1
  Derivative1/1 -> Scope1/1, thetadotdot/1
  In1/1 -> Transfer Fcn (with initial states)1/1

== system HighLevelLowLevel_Manual/Tilt Rotor Simulator/Vehicle dynamics/Arm 1/Subsystem3 ==
  In1 : Inport
  Derivative2 : Derivative
  Derivative3 : Derivative
  Scope : Scope
  Transfer Fcn (with initial states) : simulink_extras/Additional Linear/Transfer Fcn (with initial states)  N=[153.5000]  D="[1  20.06  153.3]"  X0=0
  phi : Outport
  phidot : Outport  Port=2
  phidotdot : Outport  Port=3
  wires:
  Derivative2/1 -> phidot/1, Derivative3/1
  Transfer Fcn (with initial states)/1 -> Derivative2/1, Scope/1, phi/1
  Derivative3/1 -> phidotdot/1
  In1/1 -> Transfer Fcn (with initial states)/1

== system HighLevelLowLevel_Manual/Tilt Rotor Simulator/Vehicle dynamics/Arm 2/Arm dynamics ==
  note: M = I.thetadotdot + thetadot X I.thetadot
      | followed by a conversion to body frame
  theta : Inport
  thetadot : Inport  Port=2
  thetadotdot : Inport  Port=3
  Add1 : Sum
  Cross Product1 : matrix_library/Cross Product
  Matrix Multiply2 : Product  Multiplication=Matrix(*)
  Matrix Multiply3 : Product
  Matrix Multiply4 : Product
  Matrix Multiply5 : Product  Multiplication=Matrix(*)
  Matrix Multiply6 : Product  Multiplication=Matrix(*)
  arm to body : MATLAB Function  TreatAsAtomicUnit=on
  i2 : Constant  Value=[1 ,0 ,0]'
  inertial tensor of arm : Constant  Value=[0.012 0 0; 0 0.008 0;0 0 0.019]
  M : Outport
  wires:
  Matrix Multiply3/1 -> Cross Product1/1, Matrix Multiply2/2
  inertial tensor of arm/1 -> Matrix Multiply5/1, Matrix Multiply2/1
  thetadotdot/1 -> Matrix Multiply4/1
  Matrix Multiply4/1 -> Matrix Multiply5/2
  Matrix Multiply5/1 -> Add1/2
  i2/1 -> Matrix Multiply4/2, Matrix Multiply3/2
  arm to body/1(y) -> Matrix Multiply6/1
  Matrix Multiply2/1 -> Cross Product1/2
  Cross Product1/1 -> Add1/1
  Add1/1 -> Matrix Multiply6/2
  thetadot/1 -> Matrix Multiply3/1
  Matrix Multiply6/1 -> M/1
  theta/1 -> arm to body/1(theta)

== system HighLevelLowLevel_Manual/Tilt Rotor Simulator/Vehicle dynamics/Arm 2/Prop Froces and moment ==
  note: T = Ctx w^2
      | Q = Cd x w^2
  Cd : Inport
  Ct : Inport  Port=2
  omega : Inport  Port=3
  Gain : Gain  Gain=-1
  Product{,1..3} (4 alike) : Product
  F : Outport
  M : Outport  Port=2
  wires:
  omega/1 -> Product3/1, Product2/2, Product1/2, Product/2
  Ct/1 -> Product2/1
  Product2/1 -> Product3/2
  Product3/1 -> Gain/1
  Product/1 -> Product1/1
  Product1/1 -> M/1
  Cd/1 -> Product/1
  Gain/1 -> F/1

== system HighLevelLowLevel_Manual/Tilt Rotor Simulator/Vehicle dynamics/Arm 2/Subsystem ==
  In1 : Inport
  Derivative : Derivative
  Derivative1 : Derivative
  Scope : Scope
  Transfer Fcn (with initial states)1 : simulink_extras/Additional Linear/Transfer Fcn (with initial states)  N=[153.5000]  D="[1  20.06  153.3]"  X0=0
  theta : Outport
  thetadot : Outport  Port=2
  thetadotdot : Outport  Port=3
  wires:
  Derivative/1 -> thetadot/1, Derivative1/1
  Transfer Fcn (with initial states)1/1 -> Derivative/1, Scope/1, theta/1
  Derivative1/1 -> thetadotdot/1
  In1/1 -> Transfer Fcn (with initial states)1/1

== system HighLevelLowLevel_Manual/Tilt Rotor Simulator/Vehicle dynamics/Arm 2/Subsystem1 ==
  In1 : Inport
  Derivative2 : Derivative
  Derivative3 : Derivative
  Scope : Scope
  Transfer Fcn (with initial states) : simulink_extras/Additional Linear/Transfer Fcn (with initial states)  N=[153.5000]  D="[1  20.06  153.3]"  X0=0
  phi : Outport
  phidot : Outport  Port=2
  phidotdot : Outport  Port=3
  wires:
  Derivative2/1 -> phidot/1, Derivative3/1
  Transfer Fcn (with initial states)/1 -> Derivative2/1, Scope/1, phi/1
  Derivative3/1 -> phidotdot/1
  In1/1 -> Transfer Fcn (with initial states)/1

== system HighLevelLowLevel_Manual/Tilt Rotor Simulator/Vehicle dynamics/Arm 3/Arm dynamics ==
  note: M = I.thetadotdot + thetadot X I.thetadot
      | followed by a conversion to body frame
  theta : Inport
  thetadot : Inport  Port=2
  thetadotdot : Inport  Port=3
  Add1 : Sum
  Cross Product1 : matrix_library/Cross Product
  Matrix Multiply2 : Product  Multiplication=Matrix(*)
  Matrix Multiply3 : Product
  Matrix Multiply4 : Product
  Matrix Multiply5 : Product  Multiplication=Matrix(*)
  Matrix Multiply6 : Product  Multiplication=Matrix(*)
  arm to body : MATLAB Function  TreatAsAtomicUnit=on
  i2 : Constant  Value=[1 ,0 ,0]'
  inertial tensor of arm : Constant  Value=[0.012 0 0; 0 0.008 0;0 0 0.019]
  M : Outport
  wires:
  Matrix Multiply3/1 -> Cross Product1/1, Matrix Multiply2/2
  inertial tensor of arm/1 -> Matrix Multiply5/1, Matrix Multiply2/1
  thetadotdot/1 -> Matrix Multiply4/1
  Matrix Multiply4/1 -> Matrix Multiply5/2
  Matrix Multiply5/1 -> Add1/2
  i2/1 -> Matrix Multiply4/2, Matrix Multiply3/2
  arm to body/1(y) -> Matrix Multiply6/1
  Matrix Multiply2/1 -> Cross Product1/2
  Cross Product1/1 -> Add1/1
  Add1/1 -> Matrix Multiply6/2
  thetadot/1 -> Matrix Multiply3/1
  Matrix Multiply6/1 -> M/1
  theta/1 -> arm to body/1(theta)

== system HighLevelLowLevel_Manual/Tilt Rotor Simulator/Vehicle dynamics/Arm 3/Prop Froces and moment1 ==
  note: T = Ctx w^2
      | Q = Cd x w^2
  Cd : Inport
  Ct : Inport  Port=2
  omega : Inport  Port=3
  Gain : Gain  Gain=-1
  Product{,1..3} (4 alike) : Product
  F : Outport
  M : Outport  Port=2
  wires:
  omega/1 -> Product3/1, Product2/2, Product1/2, Product/2
  Ct/1 -> Product2/1
  Product2/1 -> Product3/2
  Product3/1 -> Gain/1
  Product/1 -> Product1/1
  Product1/1 -> M/1
  Cd/1 -> Product/1
  Gain/1 -> F/1

== system HighLevelLowLevel_Manual/Tilt Rotor Simulator/Vehicle dynamics/Arm 3/Subsystem2 ==
  In1 : Inport
  Derivative : Derivative
  Derivative1 : Derivative
  Transfer Fcn (with initial states)1 : simulink_extras/Additional Linear/Transfer Fcn (with initial states)  N=[153.5000]  D="[1  20.06  153.3]"  X0=0
  theta : Outport
  thetadot : Outport  Port=2
  thetadotdot : Outport  Port=3
  wires:
  Derivative/1 -> thetadot/1, Derivative1/1
  Transfer Fcn (with initial states)1/1 -> Derivative/1, theta/1
  Derivative1/1 -> thetadotdot/1
  In1/1 -> Transfer Fcn (with initial states)1/1

== system HighLevelLowLevel_Manual/Tilt Rotor Simulator/Vehicle dynamics/Arm 3/Subsystem3 ==
  In1 : Inport
  Derivative2 : Derivative
  Derivative3 : Derivative
  Transfer Fcn (with initial states) : simulink_extras/Additional Linear/Transfer Fcn (with initial states)  N=[153.5000]  D="[1  20.06  153.3]"  X0=0
  phi : Outport
  phidot : Outport  Port=2
  phidotdot : Outport  Port=3
  wires:
  Derivative2/1 -> phidot/1, Derivative3/1
  Transfer Fcn (with initial states)/1 -> Derivative2/1, phi/1
  Derivative3/1 -> phidotdot/1
  In1/1 -> Transfer Fcn (with initial states)/1

== system HighLevelLowLevel_Manual/Tilt Rotor Simulator/Vehicle dynamics/Arm 4/Arm dynamics ==
  note: M = I.thetadotdot + thetadot X I.thetadot
      | followed by a conversion to body frame
  theta : Inport
  thetadot : Inport  Port=2
  thetadotdot : Inport  Port=3
  Add1 : Sum
  Cross Product1 : matrix_library/Cross Product
  Matrix Multiply2 : Product  Multiplication=Matrix(*)
  Matrix Multiply3 : Product
  Matrix Multiply4 : Product
  Matrix Multiply5 : Product  Multiplication=Matrix(*)
  Matrix Multiply6 : Product  Multiplication=Matrix(*)
  arm to body : MATLAB Function  TreatAsAtomicUnit=on
  i2 : Constant  Value=[1 ,0 ,0]'
  inertial tensor of arm : Constant  Value=[0.012 0 0; 0 0.008 0;0 0 0.019]
  M : Outport
  wires:
  Matrix Multiply3/1 -> Cross Product1/1, Matrix Multiply2/2
  inertial tensor of arm/1 -> Matrix Multiply5/1, Matrix Multiply2/1
  thetadotdot/1 -> Matrix Multiply4/1
  Matrix Multiply4/1 -> Matrix Multiply5/2
  Matrix Multiply5/1 -> Add1/2
  i2/1 -> Matrix Multiply4/2, Matrix Multiply3/2
  arm to body/1(y) -> Matrix Multiply6/1
  Matrix Multiply2/1 -> Cross Product1/2
  Cross Product1/1 -> Add1/1
  Add1/1 -> Matrix Multiply6/2
  thetadot/1 -> Matrix Multiply3/1
  Matrix Multiply6/1 -> M/1
  theta/1 -> arm to body/1(theta)

== system HighLevelLowLevel_Manual/Tilt Rotor Simulator/Vehicle dynamics/Arm 4/Prop Froces and moment1 ==
  note: T = Ctx w^2
      | Q = Cd x w^2
  Cd : Inport
  Ct : Inport  Port=2
  omega : Inport  Port=3
  Gain : Gain  Gain=-1
  Product{,1..3} (4 alike) : Product
  F : Outport
  M : Outport  Port=2
  wires:
  omega/1 -> Product3/1, Product2/2, Product1/2, Product/2
  Ct/1 -> Product2/1
  Product2/1 -> Product3/2
  Product3/1 -> Gain/1
  Product/1 -> Product1/1
  Product1/1 -> M/1
  Cd/1 -> Product/1
  Gain/1 -> F/1

== system HighLevelLowLevel_Manual/Tilt Rotor Simulator/Vehicle dynamics/Arm 4/Subsystem2 ==
  In1 : Inport
  Derivative : Derivative
  Derivative1 : Derivative
  Transfer Fcn (with initial states)1 : simulink_extras/Additional Linear/Transfer Fcn (with initial states)  N=[153.5000]  D="[1  20.06  153.3]"  X0=0
  theta : Outport
  thetadot : Outport  Port=2
  thetadotdot : Outport  Port=3
  wires:
  Derivative/1 -> thetadot/1, Derivative1/1
  Transfer Fcn (with initial states)1/1 -> Derivative/1, theta/1
  Derivative1/1 -> thetadotdot/1
  In1/1 -> Transfer Fcn (with initial states)1/1

== system HighLevelLowLevel_Manual/Tilt Rotor Simulator/Vehicle dynamics/Arm 4/Subsystem3 ==
  In1 : Inport
  Derivative2 : Derivative
  Derivative3 : Derivative
  Transfer Fcn (with initial states) : simulink_extras/Additional Linear/Transfer Fcn (with initial states)  N=[153.5000]  D="[1  20.06  153.3]"  X0=0
  phi : Outport
  phidot : Outport  Port=2
  phidotdot : Outport  Port=3
  wires:
  Derivative2/1 -> phidot/1, Derivative3/1
  Transfer Fcn (with initial states)/1 -> Derivative2/1, phi/1
  Derivative3/1 -> phidotdot/1
  In1/1 -> Transfer Fcn (with initial states)/1

== matlab function HighLevelLowLevel_Manual/Tilt Rotor Simulator/Vehicle dynamics/Arm 1/Arm dynamics/arm to body ==
  data: theta input; y output
function y = fcn(theta)

theta = -theta; %negating because rotation is from arm to body frame, so angle of rotation will be opposite that of that arm

y = [1 0 0;
    0 cos(theta) -sin(theta);
    0 sin(theta) cos(theta)]; %a rotation about x axis

== matlab function HighLevelLowLevel_Manual/Tilt Rotor Simulator/Vehicle dynamics/Arm 3/prop to body1 ==
  data: theta input; phi input; y output
function y = fcn(theta, phi)

y = [sin(phi); -sin(theta)*cos(phi); cos(theta)*cos(phi)]; %derived in the literature

== matlab function HighLevelLowLevel_Manual/Tilt Rotor Simulator/Vehicle dynamics/Arm 2/prop to body ==
  data: theta input; phi input; y output
function y = fcn(theta, phi)

y = [sin(phi); -sin(theta)*cos(phi); cos(theta)*cos(phi)]; %derived in the literature

== matlab function HighLevelLowLevel_Manual/Tilt Rotor Simulator/Vehicle dynamics/Arm 4/Arm dynamics/arm to body ==
  data: theta input; y output
function y = fcn(theta)

theta = -theta; %negating because rotation is from arm to body frame, so angle of rotation will be opposite that of that arm

y = [1 0 0;
    0 cos(theta) -sin(theta);
    0 sin(theta) cos(theta)]; %a rotation about x axis

== matlab function HighLevelLowLevel_Manual/Tilt Rotor Simulator/Vehicle dynamics/Arm 4/prop to body1 ==
  data: theta input; phi input; y output
function y = fcn(theta, phi)

y = [sin(phi); -sin(theta)*cos(phi); cos(theta)*cos(phi)]; %derived in the literature

== matlab function HighLevelLowLevel_Manual/Tilt Rotor Simulator/Vehicle dynamics/Arm 2/Arm dynamics/arm to body ==
  data: theta input; y output
function y = fcn(theta)

theta = -theta; %negating because rotation is from arm to body frame, so angle of rotation will be opposite that of that arm

y = [1 0 0;
    0 cos(theta) -sin(theta);
    0 sin(theta) cos(theta)]; %a rotation about x axis

== matlab function HighLevelLowLevel_Manual/Tilt Rotor Simulator/Vehicle dynamics/Arm 1/prop to body1 ==
  data: theta input; phi input; y output
function y = fcn(theta, phi)

y = [sin(phi); -sin(theta)*cos(phi); cos(theta)*cos(phi)]; %derived in the literature

== matlab function HighLevelLowLevel_Manual/Tilt Rotor Simulator/Setpoint/Manual/Deadzone ==
  data: u input; y output
function y = fcn(u)

y = zeros(size(u));
for i = 1:length(u)
    mean = 0;
    if i == 3
        mean = 0.5;
    end
    if abs(u(i) - mean) > 0.02
        y(i) = u(i);
    else
        y(i) = mean;
    end
end

== matlab function HighLevelLowLevel_Manual/Tilt Rotor Simulator/Simulated Barrier ==
  data: x input; F output; x1 parameter; x2 parameter; thickness parameter; E parameter; A parameter
function F   = wall(x, x1, x2, thickness, E, A)
    [d, direction] = point_to_line_segment_distance(x, x1, x2);
    if d <= thickness
        forceMagnitude = E * (thickness - d)/thickness * A;
        F = forceMagnitude * direction;
    else
        F = [0; 0; 0];
    end
end

function [d, direction] = point_to_line_segment_distance(x, a, b)
    ab = b - a; 
    ax = x(1:2) - a; 
    t = dot(ax, ab) / dot(ab, ab);
    t = max(0, min(1, t));
    closestPoint = a + t * ab;
    normal = [-ab(2); ab(1)];
    if dot(normal, ax) < 0
        normal = -normal;
    end
    direction = normal / norm(normal);
    direction = [direction; 0];
    d = norm(x(1:2) - closestPoint);
end

== matlab function HighLevelLowLevel_Manual/Tilt Rotor Simulator/Setpoint/Manual/MATLAB Function ==
  data: u input; max_out parameter; min_out parameter; max_in parameter; y output; min_in parameter
function y = fcn(u, max_out, min_out, max_in, min_in)

y = (max_out - min_out) / (max_in - min_in) *(u - (min_in + max_in)/2) + (max_out + min_out)/2;

== matlab function HighLevelLowLevel_Manual/Tilt Rotor Simulator/PID controller1/MATLAB Function4 ==
  data: Fz input; omega output; theta input; psi input
function omega = fcn(Fz, theta, psi)

ct= 0.00010297;

T = Fz/(cos(theta)*cos(psi));
if T >= 0
    omega = sqrt(T/ct);
else
    omega = 0;
end

== matlab function HighLevelLowLevel_Manual/Tilt Rotor Simulator/PID controller1/MATLAB Function5 ==
  data: Fz input; omega output; theta input; psi input
function omega = fcn(Fz, theta, psi)

ct= 0.00010297;

T = Fz/(cos(theta)*cos(psi));
if T >= 0
    omega = sqrt(T/ct);
else
    omega = 0;
end

== matlab function HighLevelLowLevel_Manual/Tilt Rotor Simulator/PID controller1/MATLAB Function6 ==
  data: Fz input; omega output; theta input; psi input
function omega = fcn(Fz, theta, psi)

ct= 0.00010297;

T = Fz/(cos(theta)*cos(psi));
if T >= 0
    omega = sqrt(T/ct);
else
    omega = 0;
end

== matlab function HighLevelLowLevel_Manual/Tilt Rotor Simulator/PID controller1/MATLAB Function7 ==
  data: Fz input; omega output; theta input; psi input
function omega = fcn(Fz, theta, psi)

ct= 0.00010297;

T = Fz/(cos(theta)*cos(psi));
if T >= 0
    omega = sqrt(T/ct);
else
    omega = 0;
end

== matlab function HighLevelLowLevel_Manual/Tilt Rotor Simulator/Setpoint/Manual/MATLAB Function1 ==
  data: u input; max_out parameter; min_out parameter; max_in parameter; y output; min_in parameter
function y = fcn(u, max_out, min_out, max_in, min_in)

y = (max_out - min_out) / (max_in - min_in) *(u - (min_in + max_in)/2) + (max_out + min_out)/2;

== matlab function HighLevelLowLevel_Manual/Tilt Rotor Simulator/Setpoint/Manual/MATLAB Function2 ==
  data: u input; max_out parameter; min_out parameter; max_in parameter; y output; min_in parameter
function y = fcn(u, max_out, min_out, max_in, min_in)

y = (max_out - min_out) / (max_in - min_in) *(u - (min_in + max_in)/2) + (max_out + min_out)/2;

== matlab function HighLevelLowLevel_Manual/Tilt Rotor Simulator/Setpoint/Manual/MATLAB Function3 ==
  data: u input; max_out parameter; min_out parameter; max_in parameter; y output; min_in parameter
function y = fcn(u, max_out, min_out, max_in, min_in)

y = (max_out - min_out) / (max_in - min_in) *(u - (min_in + max_in)/2) + (max_out + min_out)/2;

== matlab function HighLevelLowLevel_Manual/Tilt Rotor Simulator/controller/MATLAB Function ==
  data: gravity_correction output; Rwb input; invI parameter; l parameter; g parameter; B_t parameter
function gravity_correction  = grav_corr(Rwb, invI, l, g, B_t)

R_45 = [cosd(45) -sind(45) 0; 
        sind(45)  cosd(45) 0; 
        0         0        1];

g_body = Rwb * [0 0 6.2*g]'; %rotate gravity vector from World12 to Body12
g_term = R_45'*invI*R_45*cross([0 0 l]', g_body); %cross g_body12 with offset in body12 and multiple by I in body12
g_term = Rwb^-1*g_term; %rotate g_term from body12 to world12

G = [0;0;0;0;0;0;0;0;g;0;0;0];

gravity_correction = B_t*G;

== matlab function HighLevelLowLevel_Manual/Tilt Rotor Simulator/Setpoint/Manual/MATLAB Function4 ==
  data: u input; max_out parameter; min_out parameter; max_in parameter; y output; min_in parameter
function y = fcn(u, max_out, min_out, max_in, min_in)

y = (max_out - min_out) / (max_in - min_in) *(u - (min_in + max_in)/2) + (max_out + min_out)/2;

== matlab function HighLevelLowLevel_Manual/Tilt Rotor Simulator/Setpoint/Manual/MATLAB Function5 ==
  data: inputInt input; bitArray output; roll output; z output
function [bitArray, roll, z] = intToBitArray(inputInt)
    bitArray = zeros(1, 12);
    for i = 1:12
        bit = bitget(inputInt, i);
        bitArray(i) = bit;
    end

    roll = bitArray(6) - bitArray(5);

    z = bitArray(8) - bitArray(7); 


end

== matlab function HighLevelLowLevel_Manual/Tilt Rotor Simulator/Setpoint/Manual/MATLAB Function6 ==
  data: u input; max_out parameter; min_out parameter; max_in parameter; y output; min_in parameter
function y = fcn(u, max_out, min_out, max_in, min_in)

y = (max_out - min_out) / (max_in - min_in) *(u - (min_in + max_in)/2) + (max_out + min_out)/2;

== matlab function HighLevelLowLevel_Manual/Tilt Rotor Simulator/PID controller1/MATLAB Function1 ==
  data: F input; theta output; phi output; Fz output
function [theta, phi, Fz] = fcn(F)

f = norm(F);

theta = atan(-F(2)/F(3));

phi = asin(-F(1)/f);

Fz = -F(3);

== matlab function HighLevelLowLevel_Manual/Tilt Rotor Simulator/controller/MATLAB Function1 ==
  data: error input; y output
function y = fcn(error)

y = error;

for i= 1:length(y)
    if abs(y(i)) < .001
        y(i) = 0;
    end
end

== matlab function HighLevelLowLevel_Manual/Tilt Rotor Simulator/controller/MATLAB Function2 ==
  data: Fx input; F1 output; F2 output; F3 output; F4 output; Fy input; Fz input; M input; Rwb input
function [F1, F2, F3, F4]= F(Fx, Fy, Fz, M, Rwb)

d = 0.44;
u = [Fx;Fy;Fz;M];
R_neg45 = [cosd(45) sind(45) 0; 
        -sind(45)  cosd(45) 0; 
        0         0        1];

Frot = R_neg45 * Rwb * u(1:3); 
Mrot = R_neg45 * Rwb * u(4:6);
u_body = [Frot; Mrot]; %x aligned with prop 1

W = [1 0 0 0 1 0 -1 0 0 0 -1 0;
     0 1 0 -1 0 0 0 -1 0 1 0 0;
     0 0 1 0 0 1 0 0 1 0 0 1;
     0 0 0 0 0 -d 0 0 0 0 0 d;
     0 0 -d 0 0 0 0 0 d 0 0 0;
     0 d 0 0 d 0 0 d 0 0 d 0]; % u_body = W * F

W_t = pinv(W); 

if u(3) <= 0 
    u(3) = 0;
end

F_props = W_t*u_body;  %inividual prop forces each in their own frames

F1 = F_props(1:3); 
F2 = F_props(4:6);
F3 = F_props(7:9); 
F4 = F_props(10:12);

== matlab function HighLevelLowLevel_Manual/Tilt Rotor Simulator/PID controller1/MATLAB Function ==
  data: F input; theta output; phi output; Fz output
function [theta, phi, Fz] = fcn(F)

f = norm(F);

theta = atan(-F(2)/F(3));

phi = asin(-F(1)/f);

Fz = -F(3);

== matlab function HighLevelLowLevel_Manual/Tilt Rotor Simulator/PID controller1/MATLAB Function2 ==
  data: F input; theta output; phi output; Fz output
function [theta, phi, Fz] = fcn(F)

f = norm(F);

theta = atan(-F(2)/F(3));

phi = asin(-F(1)/f);

Fz = -F(3);

== matlab function HighLevelLowLevel_Manual/Tilt Rotor Simulator/PID controller1/MATLAB Function3 ==
  data: F input; theta output; phi output; Fz output
function [theta, phi, Fz] = fcn(F)

f = norm(F);

theta = atan(-F(2)/F(3));

phi = asin(-F(1)/f);

Fz = -F(3);

== matlab function HighLevelLowLevel_Manual/Tilt Rotor Simulator/Vehicle dynamics/Arm 3/Arm dynamics/arm to body ==
  data: theta input; y output
function y = fcn(theta)

theta = -theta; %negating because rotation is from arm to body frame, so angle of rotation will be opposite that of that arm

y = [1 0 0;
    0 cos(theta) -sin(theta);
    0 sin(theta) cos(theta)]; %a rotation about x axis
